simulink model "RFID"  (R2023a)
settings: Solver=VariableStepAuto  StartTime=0.0  StopTime=10.0  RelTol=1e-3
(part 1 of 2)
settings Model: Creator=SESA710169  LastModifiedBy=SESA710169

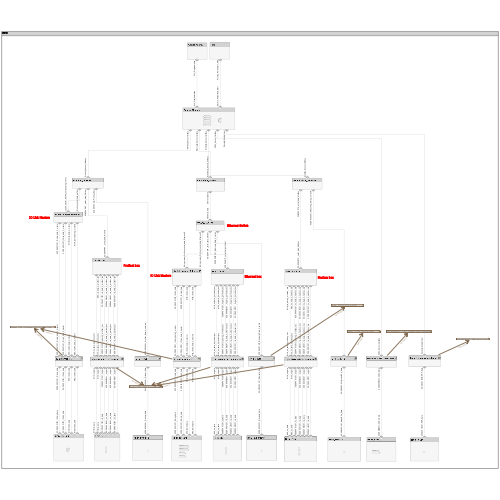
[thumbnail: Simulink's stored preview of the top-level diagram]
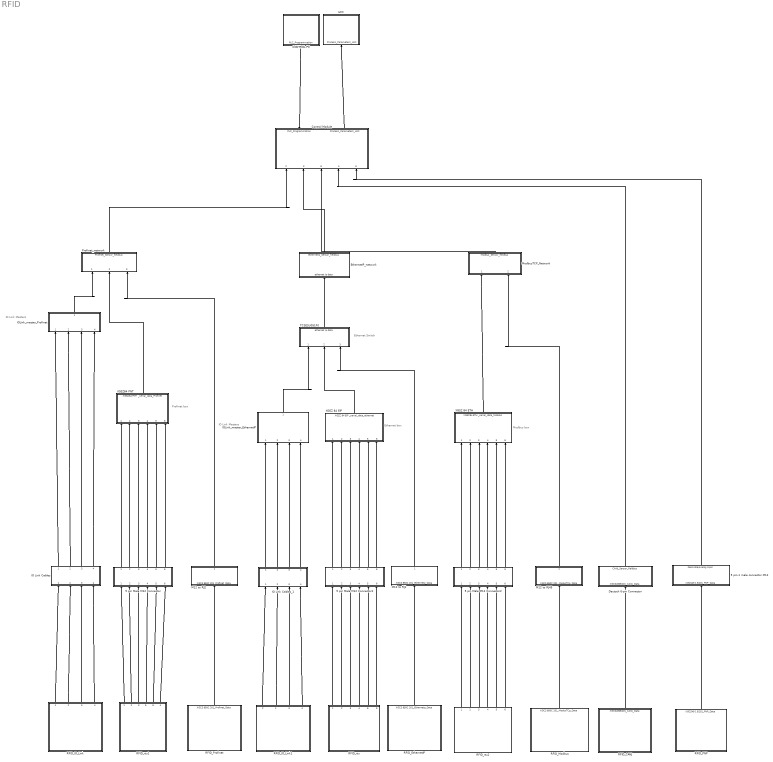
== system RFID ==
  note: IO Link Masters
  note: Modbus box
  note: Ethernet Switch
  note: Ethernet box
  note: IO Link Masters
  note: Profinet box
  5 pin Male M12 Connector : Subsystem
      settings: PortSchema="{\"entries\":[{\"content\":{\"headerSize\":26,\"margin\":15,\"minimumSpacing\":25,\"sides\":[{\"content\":{},\"type\":\"ConnectorPlacement.EquallySpacedRectSide\",\"uuid\":\"15872914-72ca-49c0-af57-e7ce3a34352d\"},{\"content\":{\"side\":\"RIGHT\"},\"type\":\"ConnectorPlacement.EquallySpacedRectSide\",\"uuid\":\"e1987595-5073-4cb0-bc3a-ce3e48eeeb38\"},{\"content\":{\"connectorIds\":[\"Out1\",\"Out2\",\"Out3\",\"Out4\",\"Out5\",\"Out6\"],\"side\":\"TOP\"},\"type\":\"ConnectorPlacement.EquallySpacedRectSide\",\"uuid\":\"34465e36-1a4b-47f4-80e2-40bdf2aa77c4\"},{\"content\":{\"connectorIds\":[\"In1\",\"In2\",\"In3\",\"In4\",\"In5\",\"In6\"],\"side\":\"BOTTOM\"},\"type\":\"ConnectorPlacement.EquallySpacedRectSide\",\"uuid\":\"7ee8196c-d26c-4fad-bba2-16755bce26d2\"}]},\"type\":\"ConnectorPlacement.EquallySpacedConnector\",\"uuid\":\"ac1f4730-dff7-48b7-9147-a46c79733028\"}],\"packageUris\":[\"http://schema.mathworks.com/mf0/Connector/R2020b\"],\"version\":\"1.0\"}"
  5 pin Male M12 Connector1 : Subsystem
      settings: PortSchema="{\"entries\":[{\"content\":{\"headerSize\":26,\"margin\":15,\"minimumSpacing\":25,\"sides\":[{\"content\":{},\"type\":\"ConnectorPlacement.EquallySpacedRectSide\",\"uuid\":\"15872914-72ca-49c0-af57-e7ce3a34352d\"},{\"content\":{\"side\":\"RIGHT\"},\"type\":\"ConnectorPlacement.EquallySpacedRectSide\",\"uuid\":\"e1987595-5073-4cb0-bc3a-ce3e48eeeb38\"},{\"content\":{\"connectorIds\":[\"Out1\",\"Out2\",\"Out3\",\"Out4\",\"Out5\",\"Out6\"],\"side\":\"TOP\"},\"type\":\"ConnectorPlacement.EquallySpacedRectSide\",\"uuid\":\"34465e36-1a4b-47f4-80e2-40bdf2aa77c4\"},{\"content\":{\"connectorIds\":[\"In1\",\"In2\",\"In3\",\"In4\",\"In5\",\"In6\"],\"side\":\"BOTTOM\"},\"type\":\"ConnectorPlacement.EquallySpacedRectSide\",\"uuid\":\"7ee8196c-d26c-4fad-bba2-16755bce26d2\"}]},\"type\":\"ConnectorPlacement.EquallySpacedConnector\",\"uuid\":\"ac1f4730-dff7-48b7-9147-a46c79733028\"}],\"packageUris\":[\"http://schema.mathworks.com/mf0/Connector/R2020b\"],\"version\":\"1.0\"}"
  5 pin Male M12 Connector2 : Subsystem
      settings: PortSchema="{\"entries\":[{\"content\":{\"headerSize\":26,\"margin\":15,\"minimumSpacing\":25,\"sides\":[{\"content\":{},\"type\":\"ConnectorPlacement.EquallySpacedRectSide\",\"uuid\":\"15872914-72ca-49c0-af57-e7ce3a34352d\"},{\"content\":{\"side\":\"RIGHT\"},\"type\":\"ConnectorPlacement.EquallySpacedRectSide\",\"uuid\":\"e1987595-5073-4cb0-bc3a-ce3e48eeeb38\"},{\"content\":{\"connectorIds\":[\"Out1\",\"Out2\",\"Out3\",\"Out4\",\"Out5\",\"Out6\"],\"side\":\"TOP\"},\"type\":\"ConnectorPlacement.EquallySpacedRectSide\",\"uuid\":\"34465e36-1a4b-47f4-80e2-40bdf2aa77c4\"},{\"content\":{\"connectorIds\":[\"In1\",\"In2\",\"In3\",\"In4\",\"In5\",\"In6\"],\"side\":\"BOTTOM\"},\"type\":\"ConnectorPlacement.EquallySpacedRectSide\",\"uuid\":\"7ee8196c-d26c-4fad-bba2-16755bce26d2\"}]},\"type\":\"ConnectorPlacement.EquallySpacedConnector\",\"uuid\":\"ac1f4730-dff7-48b7-9147-a46c79733028\"}],\"packageUris\":[\"http://schema.mathworks.com/mf0/Connector/R2020b\"],\"version\":\"1.0\"}"
  5 pin-1 male connector M12 : Subsystem
      settings: PortSchema="{\"entries\":[{\"content\":{\"headerSize\":26,\"margin\":15,\"minimumSpacing\":25,\"sides\":[{\"content\":{},\"type\":\"ConnectorPlacement.EquallySpacedRectSide\",\"uuid\":\"fd0e21b1-4690-476b-bc14-5c8fc71147f2\"},{\"content\":{\"side\":\"RIGHT\"},\"type\":\"ConnectorPlacement.EquallySpacedRectSide\",\"uuid\":\"81f5b1ef-d6a4-481c-8562-3dd4bbf12531\"},{\"content\":{\"connectorIds\":[\"Out1\"],\"side\":\"TOP\"},\"type\":\"ConnectorPlacement.EquallySpacedRectSide\",\"uuid\":\"ad97ad28-8845-419a-93af-6ade5c0bdfbe\"},{\"content\":{\"connectorIds\":[\"In1\"],\"side\":\"BOTTOM\"},\"type\":\"ConnectorPlacement.EquallySpacedRectSide\",\"uuid\":\"20c3ec93-f654-4080-81db-cffef7cb2cf6\"}]},\"type\":\"ConnectorPlacement.EquallySpacedConnector\",\"uuid\":\"3726fd7c-4b1c-4d15-a99a-e883e4d72662\"}],\"packageUris\":[\"http://schema.mathworks.com/mf0/Connector/R2020b\"],\"version\":\"1.0\"}"
  CONTROL PC : Subsystem
      settings: PortSchema="{\"entries\":[{\"content\":{\"headerSize\":26,\"margin\":15,\"minimumSpacing\":25,\"sides\":[{\"content\":{},\"type\":\"ConnectorPlacement.EquallySpacedRectSide\",\"uuid\":\"ff8f3bf2-d6f6-4ecc-9677-a0e5f5ade440\"},{\"content\":{\"side\":\"RIGHT\"},\"type\":\"ConnectorPlacement.EquallySpacedRectSide\",\"uuid\":\"fe155757-f3d5-40d8-a583-dbbc24843437\"},{\"content\":{\"side\":\"TOP\"},\"type\":\"ConnectorPlacement.EquallySpacedRectSide\",\"uuid\":\"51bc4fd0-0675-45de-93bd-0dc8d94c5489\"},{\"content\":{\"connectorIds\":[\"Out1\"],\"side\":\"BOTTOM\"},\"type\":\"ConnectorPlacement.EquallySpacedRectSide\",\"uuid\":\"d1c979f7-175f-4276-8069-5d6ac2f759ac\"}]},\"type\":\"ConnectorPlacement.EquallySpacedConnector\",\"uuid\":\"7eb8fdf8-dbe2-49f3-b9bd-384f85dcc997\"}],\"packageUris\":[\"http://schema.mathworks.com/mf0/Connector/R2020b\"],\"version\":\"1.0\"}"
  Control Module : Subsystem
      settings: PortSchema="{\"entries\":[{\"content\":{\"headerSize\":26,\"margin\":15,\"minimumSpacing\":25,\"sides\":[{\"content\":{},\"type\":\"ConnectorPlacement.EquallySpacedRectSide\",\"uuid\":\"1d52692e-0f44-4113-9236-a25bdb619ad6\"},{\"content\":{\"side\":\"RIGHT\"},\"type\":\"ConnectorPlacement.EquallySpacedRectSide\",\"uuid\":\"ebd7129d-6295-43a2-a8fa-ceade73e4712\"},{\"content\":{\"connectorIds\":[\"In1\",\"Out1\"],\"side\":\"TOP\"},\"type\":\"ConnectorPlacement.EquallySpacedRectSide\",\"uuid\":\"449c4e30-53b6-483f-ab84-235a0572996a\"},{\"content\":{\"connectorIds\":[\"In2\",\"In3\",\"In6\",\"In4\",\"In5\"],\"side\":\"BOTTOM\"},\"type\":\"ConnectorPlacement.EquallySpacedRectSide\",\"uuid\":\"9ddc23bf-eea9-4734-a916-f94a55c11bfe\"}]},\"type\":\"ConnectorPlacement.EquallySpacedConnector\",\"uuid\":\"d9df497a-181c-43b5-b6eb-3f69da1cdffc\"}],\"packageUris\":[\"http://schema.mathworks.com/mf0/Connector/R2020b\"],\"version\":\"1.0\"}"
  Deutsch 6-pin Connector : Subsystem
      settings: PortSchema="{\"entries\":[{\"content\":{\"headerSize\":26,\"margin\":15,\"minimumSpacing\":25,\"sides\":[{\"content\":{},\"type\":\"ConnectorPlacement.EquallySpacedRectSide\",\"uuid\":\"fd0e21b1-4690-476b-bc14-5c8fc71147f2\"},{\"content\":{\"side\":\"RIGHT\"},\"type\":\"ConnectorPlacement.EquallySpacedRectSide\",\"uuid\":\"81f5b1ef-d6a4-481c-8562-3dd4bbf12531\"},{\"content\":{\"connectorIds\":[\"Out1\"],\"side\":\"TOP\"},\"type\":\"ConnectorPlacement.EquallySpacedRectSide\",\"uuid\":\"ad97ad28-8845-419a-93af-6ade5c0bdfbe\"},{\"content\":{\"connectorIds\":[\"In1\"],\"side\":\"BOTTOM\"},\"type\":\"ConnectorPlacement.EquallySpacedRectSide\",\"uuid\":\"6cb1918c-498c-482e-975f-fc177a7f5f38\"}]},\"type\":\"ConnectorPlacement.EquallySpacedConnector\",\"uuid\":\"3726fd7c-4b1c-4d15-a99a-e883e4d72662\"}],\"packageUris\":[\"http://schema.mathworks.com/mf0/Connector/R2020b\"],\"version\":\"1.0\"}"
  EthernetIP_network : Subsystem
      settings: PortSchema="{\"entries\":[{\"content\":{\"headerSize\":26,\"margin\":15,\"minimumSpacing\":25,\"sides\":[{\"content\":{},\"type\":\"ConnectorPlacement.EquallySpacedRectSide\",\"uuid\":\"ff8f3bf2-d6f6-4ecc-9677-a0e5f5ade440\"},{\"content\":{\"side\":\"RIGHT\"},\"type\":\"ConnectorPlacement.EquallySpacedRectSide\",\"uuid\":\"fe155757-f3d5-40d8-a583-dbbc24843437\"},{\"content\":{\"connectorIds\":[\"Out1\"],\"side\":\"TOP\"},\"type\":\"ConnectorPlacement.EquallySpacedRectSide\",\"uuid\":\"51bc4fd0-0675-45de-93bd-0dc8d94c5489\"},{\"content\":{\"connectorIds\":[\"In1\"],\"side\":\"BOTTOM\"},\"type\":\"ConnectorPlacement.EquallySpacedRectSide\",\"uuid\":\"a6a48096-45e8-4078-827c-8af3dc9f1ee5\"}]},\"type\":\"ConnectorPlacement.EquallySpacedConnector\",\"uuid\":\"7eb8fdf8-dbe2-49f3-b9bd-384f85dcc997\"}],\"packageUris\":[\"http://schema.mathworks.com/mf0/Connector/R2020b\"],\"version\":\"1.0\"}"
  HMI : Subsystem
      settings: PortSchema="{\"entries\":[{\"content\":{\"headerSize\":26,\"margin\":15,\"minimumSpacing\":25,\"sides\":[{\"content\":{},\"type\":\"ConnectorPlacement.EquallySpacedRectSide\",\"uuid\":\"ff8f3bf2-d6f6-4ecc-9677-a0e5f5ade440\"},{\"content\":{\"side\":\"RIGHT\"},\"type\":\"ConnectorPlacement.EquallySpacedRectSide\",\"uuid\":\"fe155757-f3d5-40d8-a583-dbbc24843437\"},{\"content\":{\"side\":\"TOP\"},\"type\":\"ConnectorPlacement.EquallySpacedRectSide\",\"uuid\":\"51bc4fd0-0675-45de-93bd-0dc8d94c5489\"},{\"content\":{\"connectorIds\":[\"In1\"],\"side\":\"BOTTOM\"},\"type\":\"ConnectorPlacement.EquallySpacedRectSide\",\"uuid\":\"52c645db-393c-4514-a828-b3b130807567\"}]},\"type\":\"ConnectorPlacement.EquallySpacedConnector\",\"uuid\":\"7eb8fdf8-dbe2-49f3-b9bd-384f85dcc997\"}],\"packageUris\":[\"http://schema.mathworks.com/mf0/Connector/R2020b\"],\"version\":\"1.0\"}"
  IO Link Cables : Subsystem
      settings: PortSchema="{\"entries\":[{\"content\":{\"headerSize\":26,\"margin\":15,\"minimumSpacing\":25,\"sides\":[{\"content\":{},\"type\":\"ConnectorPlacement.EquallySpacedRectSide\",\"uuid\":\"114e0369-1e7a-4a46-bf9a-9a919302ecfe\"},{\"content\":{\"side\":\"RIGHT\"},\"type\":\"ConnectorPlacement.EquallySpacedRectSide\",\"uuid\":\"b401c2e5-2b5e-49de-abeb-2a7da0ded51e\"},{\"content\":{\"connectorIds\":[\"Out1\",\"Out2\",\"Out3\",\"Out4\"],\"side\":\"TOP\"},\"type\":\"ConnectorPlacement.EquallySpacedRectSide\",\"uuid\":\"300c240b-1dd5-4827-92ce-421815ba1fec\"},{\"content\":{\"connectorIds\":[\"In1\",\"In2\",\"In3\",\"In4\"],\"side\":\"BOTTOM\"},\"type\":\"ConnectorPlacement.EquallySpacedRectSide\",\"uuid\":\"4925845a-f056-46c0-9ec5-2efc31482337\"}]},\"type\":\"ConnectorPlacement.EquallySpacedConnector\",\"uuid\":\"3ba3c251-a23f-40e6-ae10-3e1f576377ed\"}],\"packageUris\":[\"http://schema.mathworks.com/mf0/Connector/R2020b\"],\"version\":\"1.0\"}"
  IO Link Cables_1 : Subsystem
      settings: PortSchema="{\"entries\":[{\"content\":{\"headerSize\":26,\"margin\":15,\"minimumSpacing\":25,\"sides\":[{\"content\":{},\"type\":\"ConnectorPlacement.EquallySpacedRectSide\",\"uuid\":\"114e0369-1e7a-4a46-bf9a-9a919302ecfe\"},{\"content\":{\"side\":\"RIGHT\"},\"type\":\"ConnectorPlacement.EquallySpacedRectSide\",\"uuid\":\"b401c2e5-2b5e-49de-abeb-2a7da0ded51e\"},{\"content\":{\"connectorIds\":[\"Out1\",\"Out2\",\"Out3\",\"Out4\"],\"side\":\"TOP\"},\"type\":\"ConnectorPlacement.EquallySpacedRectSide\",\"uuid\":\"300c240b-1dd5-4827-92ce-421815ba1fec\"},{\"content\":{\"connectorIds\":[\"In1\",\"In2\",\"In3\",\"In4\"],\"side\":\"BOTTOM\"},\"type\":\"ConnectorPlacement.EquallySpacedRectSide\",\"uuid\":\"4925845a-f056-46c0-9ec5-2efc31482337\"}]},\"type\":\"ConnectorPlacement.EquallySpacedConnector\",\"uuid\":\"3ba3c251-a23f-40e6-ae10-3e1f576377ed\"}],\"packageUris\":[\"http://schema.mathworks.com/mf0/Connector/R2020b\"],\"version\":\"1.0\"}"
  IOLink_master_EthernetIP : Subsystem
      settings: PortSchema="{\"entries\":[{\"content\":{\"headerSize\":26,\"margin\":15,\"minimumSpacing\":25,\"sides\":[{\"content\":{},\"type\":\"ConnectorPlacement.EquallySpacedRectSide\",\"uuid\":\"ff8f3bf2-d6f6-4ecc-9677-a0e5f5ade440\"},{\"content\":{\"side\":\"RIGHT\"},\"type\":\"ConnectorPlacement.EquallySpacedRectSide\",\"uuid\":\"fe155757-f3d5-40d8-a583-dbbc24843437\"},{\"content\":{\"connectorIds\":[\"Out1\"],\"side\":\"TOP\"},\"type\":\"ConnectorPlacement.EquallySpacedRectSide\",\"uuid\":\"51bc4fd0-0675-45de-93bd-0dc8d94c5489\"},{\"content\":{\"connectorIds\":[\"In1\",\"In2\",\"In3\",\"In4\"],\"side\":\"BOTTOM\"},\"type\":\"ConnectorPlacement.EquallySpacedRectSide\",\"uuid\":\"96d1ea42-fb86-44af-b869-0fda48dfe9a2\"}]},\"type\":\"ConnectorPlacement.EquallySpacedConnector\",\"uuid\":\"7eb8fdf8-dbe2-49f3-b9bd-384f85dcc997\"}],\"packageUris\":[\"http://schema.mathworks.com/mf0/Connector/R2020b\"],\"version\":\"1.0\"}"
  IOLink_master_Profinet : Subsystem
      settings: PortSchema="{\"entries\":[{\"content\":{\"headerSize\":26,\"margin\":15,\"minimumSpacing\":25,\"sides\":[{\"content\":{},\"type\":\"ConnectorPlacement.EquallySpacedRectSide\",\"uuid\":\"ff8f3bf2-d6f6-4ecc-9677-a0e5f5ade440\"},{\"content\":{\"side\":\"RIGHT\"},\"type\":\"ConnectorPlacement.EquallySpacedRectSide\",\"uuid\":\"fe155757-f3d5-40d8-a583-dbbc24843437\"},{\"content\":{\"connectorIds\":[\"Out1\"],\"side\":\"TOP\"},\"type\":\"ConnectorPlacement.EquallySpacedRectSide\",\"uuid\":\"51bc4fd0-0675-45de-93bd-0dc8d94c5489\"},{\"content\":{\"connectorIds\":[\"In1\",\"In2\",\"In3\",\"In4\"],\"side\":\"BOTTOM\"},\"type\":\"ConnectorPlacement.EquallySpacedRectSide\",\"uuid\":\"96d1ea42-fb86-44af-b869-0fda48dfe9a2\"}]},\"type\":\"ConnectorPlacement.EquallySpacedConnector\",\"uuid\":\"7eb8fdf8-dbe2-49f3-b9bd-384f85dcc997\"}],\"packageUris\":[\"http://schema.mathworks.com/mf0/Connector/R2020b\"],\"version\":\"1.0\"}"
  M12 to RJ1 : Subsystem
      settings: PortSchema="{\"entries\":[{\"content\":{\"headerSize\":26,\"margin\":15,\"minimumSpacing\":25,\"sides\":[{\"content\":{},\"type\":\"ConnectorPlacement.EquallySpacedRectSide\",\"uuid\":\"15872914-72ca-49c0-af57-e7ce3a34352d\"},{\"content\":{\"side\":\"RIGHT\"},\"type\":\"ConnectorPlacement.EquallySpacedRectSide\",\"uuid\":\"e1987595-5073-4cb0-bc3a-ce3e48eeeb38\"},{\"content\":{\"connectorIds\":[\"Out1\"],\"side\":\"TOP\"},\"type\":\"ConnectorPlacement.EquallySpacedRectSide\",\"uuid\":\"34465e36-1a4b-47f4-80e2-40bdf2aa77c4\"},{\"content\":{\"connectorIds\":[\"In1\"],\"side\":\"BOTTOM\"},\"type\":\"ConnectorPlacement.EquallySpacedRectSide\",\"uuid\":\"232f6760-6a21-49f2-ae01-222b23a991b9\"}]},\"type\":\"ConnectorPlacement.EquallySpacedConnector\",\"uuid\":\"ac1f4730-dff7-48b7-9147-a46c79733028\"}],\"packageUris\":[\"http://schema.mathworks.com/mf0/Connector/R2020b\"],\"version\":\"1.0\"}"
  M12 to RJ2 : Subsystem
      settings: PortSchema="{\"entries\":[{\"content\":{\"headerSize\":26,\"margin\":15,\"minimumSpacing\":25,\"sides\":[{\"content\":{},\"type\":\"ConnectorPlacement.EquallySpacedRectSide\",\"uuid\":\"15872914-72ca-49c0-af57-e7ce3a34352d\"},{\"content\":{\"side\":\"RIGHT\"},\"type\":\"ConnectorPlacement.EquallySpacedRectSide\",\"uuid\":\"e1987595-5073-4cb0-bc3a-ce3e48eeeb38\"},{\"content\":{\"connectorIds\":[\"Out1\"],\"side\":\"TOP\"},\"type\":\"ConnectorPlacement.EquallySpacedRectSide\",\"uuid\":\"34465e36-1a4b-47f4-80e2-40bdf2aa77c4\"},{\"content\":{\"connectorIds\":[\"In1\"],\"side\":\"BOTTOM\"},\"type\":\"ConnectorPlacement.EquallySpacedRectSide\",\"uuid\":\"232f6760-6a21-49f2-ae01-222b23a991b9\"}]},\"type\":\"ConnectorPlacement.EquallySpacedConnector\",\"uuid\":\"ac1f4730-dff7-48b7-9147-a46c79733028\"}],\"packageUris\":[\"http://schema.mathworks.com/mf0/Connector/R2020b\"],\"version\":\"1.0\"}"
  M12 to RJ45 : Subsystem
      settings: PortSchema="{\"entries\":[{\"content\":{\"headerSize\":26,\"margin\":15,\"minimumSpacing\":25,\"sides\":[{\"content\":{},\"type\":\"ConnectorPlacement.EquallySpacedRectSide\",\"uuid\":\"15872914-72ca-49c0-af57-e7ce3a34352d\"},{\"content\":{\"side\":\"RIGHT\"},\"type\":\"ConnectorPlacement.EquallySpacedRectSide\",\"uuid\":\"e1987595-5073-4cb0-bc3a-ce3e48eeeb38\"},{\"content\":{\"connectorIds\":[\"Out1\"],\"side\":\"TOP\"},\"type\":\"ConnectorPlacement.EquallySpacedRectSide\",\"uuid\":\"34465e36-1a4b-47f4-80e2-40bdf2aa77c4\"},{\"content\":{\"connectorIds\":[\"In1\"],\"side\":\"BOTTOM\"},\"type\":\"ConnectorPlacement.EquallySpacedRectSide\",\"uuid\":\"232f6760-6a21-49f2-ae01-222b23a991b9\"}]},\"type\":\"ConnectorPlacement.EquallySpacedConnector\",\"uuid\":\"ac1f4730-dff7-48b7-9147-a46c79733028\"}],\"packageUris\":[\"http://schema.mathworks.com/mf0/Connector/R2020b\"],\"version\":\"1.0\"}"
  ModbusTCP_Network : Subsystem
      settings: PortSchema="{\"entries\":[{\"content\":{\"headerSize\":26,\"margin\":15,\"minimumSpacing\":25,\"sides\":[{\"content\":{},\"type\":\"ConnectorPlacement.EquallySpacedRectSide\",\"uuid\":\"ff8f3bf2-d6f6-4ecc-9677-a0e5f5ade440\"},{\"content\":{\"side\":\"RIGHT\"},\"type\":\"ConnectorPlacement.EquallySpacedRectSide\",\"uuid\":\"fe155757-f3d5-40d8-a583-dbbc24843437\"},{\"content\":{\"connectorIds\":[\"Out1\"],\"side\":\"TOP\"},\"type\":\"ConnectorPlacement.EquallySpacedRectSide\",\"uuid\":\"51bc4fd0-0675-45de-93bd-0dc8d94c5489\"},{\"content\":{\"connectorIds\":[\"In1\",\"In2\"],\"side\":\"BOTTOM\"},\"type\":\"ConnectorPlacement.EquallySpacedRectSide\",\"uuid\":\"a6a48096-45e8-4078-827c-8af3dc9f1ee5\"}]},\"type\":\"ConnectorPlacement.EquallySpacedConnector\",\"uuid\":\"7eb8fdf8-dbe2-49f3-b9bd-384f85dcc997\"}],\"packageUris\":[\"http://schema.mathworks.com/mf0/Connector/R2020b\"],\"version\":\"1.0\"}"
  Profinet_network : Subsystem
      settings: PortSchema="{\"entries\":[{\"content\":{\"headerSize\":26,\"margin\":15,\"minimumSpacing\":25,\"sides\":[{\"content\":{},\"type\":\"ConnectorPlacement.EquallySpacedRectSide\",\"uuid\":\"ff8f3bf2-d6f6-4ecc-9677-a0e5f5ade440\"},{\"content\":{\"side\":\"RIGHT\"},\"type\":\"ConnectorPlacement.EquallySpacedRectSide\",\"uuid\":\"fe155757-f3d5-40d8-a583-dbbc24843437\"},{\"content\":{\"connectorIds\":[\"Out1\"],\"side\":\"TOP\"},\"type\":\"ConnectorPlacement.EquallySpacedRectSide\",\"uuid\":\"51bc4fd0-0675-45de-93bd-0dc8d94c5489\"},{\"content\":{\"connectorIds\":[\"In1\",\"In2\",\"In3\"],\"side\":\"BOTTOM\"},\"type\":\"ConnectorPlacement.EquallySpacedRectSide\",\"uuid\":\"a6a48096-45e8-4078-827c-8af3dc9f1ee5\"}]},\"type\":\"ConnectorPlacement.EquallySpacedConnector\",\"uuid\":\"7eb8fdf8-dbe2-49f3-b9bd-384f85dcc997\"}],\"packageUris\":[\"http://schema.mathworks.com/mf0/Connector/R2020b\"],\"version\":\"1.0\"}"
  RFID_CANJ : Subsystem
      settings: PortSchema="{\"entries\":[{\"content\":{\"headerSize\":26,\"margin\":15,\"minimumSpacing\":25,\"sides\":[{\"content\":{},\"type\":\"ConnectorPlacement.EquallySpacedRectSide\",\"uuid\":\"e0eb1e50-4962-459a-8fec-1c017d32fce9\"},{\"content\":{\"side\":\"RIGHT\"},\"type\":\"ConnectorPlacement.EquallySpacedRectSide\",\"uuid\":\"13b866c0-40d0-4daf-b8cf-e6d1decf5d11\"},{\"content\":{\"connectorIds\":[\"Out1\"],\"side\":\"TOP\"},\"type\":\"ConnectorPlacement.EquallySpacedRectSide\",\"uuid\":\"2f503909-3154-427d-b557-3b7bc001611f\"}]},\"type\":\"ConnectorPlacement.EquallySpacedConnector\",\"uuid\":\"e4954000-e918-49fc-93eb-b443de9c48d9\"}],\"packageUris\":[\"http://schema.mathworks.com/mf0/Connector/R2020b\"],\"version\":\"1.0\"}"
  RFID_EthernetIP : Subsystem
      settings: PortSchema="{\"entries\":[{\"content\":{\"headerSize\":26,\"margin\":15,\"minimumSpacing\":25,\"sides\":[{\"content\":{},\"type\":\"ConnectorPlacement.EquallySpacedRectSide\",\"uuid\":\"e0eb1e50-4962-459a-8fec-1c017d32fce9\"},{\"content\":{\"side\":\"RIGHT\"},\"type\":\"ConnectorPlacement.EquallySpacedRectSide\",\"uuid\":\"13b866c0-40d0-4daf-b8cf-e6d1decf5d11\"},{\"content\":{\"connectorIds\":[\"Out1\"],\"side\":\"TOP\"},\"type\":\"ConnectorPlacement.EquallySpacedRectSide\",\"uuid\":\"2f503909-3154-427d-b557-3b7bc001611f\"}]},\"type\":\"ConnectorPlacement.EquallySpacedConnector\",\"uuid\":\"e4954000-e918-49fc-93eb-b443de9c48d9\"}],\"packageUris\":[\"http://schema.mathworks.com/mf0/Connector/R2020b\"],\"version\":\"1.0\"}"
  RFID_IO_Link : Subsystem
      settings: PortSchema="{\"entries\":[{\"content\":{\"headerSize\":26,\"margin\":15,\"minimumSpacing\":25,\"sides\":[{\"content\":{},\"type\":\"ConnectorPlacement.EquallySpacedRectSide\",\"uuid\":\"ff8f3bf2-d6f6-4ecc-9677-a0e5f5ade440\"},{\"content\":{\"side\":\"RIGHT\"},\"type\":\"ConnectorPlacement.EquallySpacedRectSide\",\"uuid\":\"fe155757-f3d5-40d8-a583-dbbc24843437\"},{\"content\":{\"connectorIds\":[\"Out1\",\"Out2\",\"Out3\",\"Out4\"],\"side\":\"TOP\"},\"type\":\"ConnectorPlacement.EquallySpacedRectSide\",\"uuid\":\"51bc4fd0-0675-45de-93bd-0dc8d94c5489\"}]},\"type\":\"ConnectorPlacement.EquallySpacedConnector\",\"uuid\":\"7eb8fdf8-dbe2-49f3-b9bd-384f85dcc997\"}],\"packageUris\":[\"http://schema.mathworks.com/mf0/Connector/R2020b\"],\"version\":\"1.0\"}"
  RFID_IO_Link1 : Subsystem
      settings: PortSchema="{\"entries\":[{\"content\":{\"headerSize\":26,\"margin\":15,\"minimumSpacing\":25,\"sides\":[{\"content\":{},\"type\":\"ConnectorPlacement.EquallySpacedRectSide\",\"uuid\":\"ff8f3bf2-d6f6-4ecc-9677-a0e5f5ade440\"},{\"content\":{\"side\":\"RIGHT\"},\"type\":\"ConnectorPlacement.EquallySpacedRectSide\",\"uuid\":\"fe155757-f3d5-40d8-a583-dbbc24843437\"},{\"content\":{\"connectorIds\":[\"Out2\",\"Out1\",\"Out3\",\"Out4\"],\"side\":\"TOP\"},\"type\":\"ConnectorPlacement.EquallySpacedRectSide\",\"uuid\":\"51bc4fd0-0675-45de-93bd-0dc8d94c5489\"}]},\"type\":\"ConnectorPlacement.EquallySpacedConnector\",\"uuid\":\"7eb8fdf8-dbe2-49f3-b9bd-384f85dcc997\"}],\"packageUris\":[\"http://schema.mathworks.com/mf0/Connector/R2020b\"],\"version\":\"1.0\"}"
  RFID_Modbus : Subsystem
      settings: PortSchema="{\"entries\":[{\"content\":{\"headerSize\":26,\"margin\":15,\"minimumSpacing\":25,\"sides\":[{\"content\":{},\"type\":\"ConnectorPlacement.EquallySpacedRectSide\",\"uuid\":\"e0eb1e50-4962-459a-8fec-1c017d32fce9\"},{\"content\":{\"side\":\"RIGHT\"},\"type\":\"ConnectorPlacement.EquallySpacedRectSide\",\"uuid\":\"13b866c0-40d0-4daf-b8cf-e6d1decf5d11\"},{\"content\":{\"connectorIds\":[\"Out1\"],\"side\":\"TOP\"},\"type\":\"ConnectorPlacement.EquallySpacedRectSide\",\"uuid\":\"2f503909-3154-427d-b557-3b7bc001611f\"}]},\"type\":\"ConnectorPlacement.EquallySpacedConnector\",\"uuid\":\"e4954000-e918-49fc-93eb-b443de9c48d9\"}],\"packageUris\":[\"http://schema.mathworks.com/mf0/Connector/R2020b\"],\"version\":\"1.0\"}"
  RFID_PNP : Subsystem
      settings: PortSchema="{\"entries\":[{\"content\":{\"headerSize\":26,\"margin\":15,\"minimumSpacing\":25,\"sides\":[{\"content\":{},\"type\":\"ConnectorPlacement.EquallySpacedRectSide\",\"uuid\":\"e0eb1e50-4962-459a-8fec-1c017d32fce9\"},{\"content\":{\"side\":\"RIGHT\"},\"type\":\"ConnectorPlacement.EquallySpacedRectSide\",\"uuid\":\"13b866c0-40d0-4daf-b8cf-e6d1decf5d11\"},{\"content\":{\"connectorIds\":[\"Out1\"],\"side\":\"TOP\"},\"type\":\"ConnectorPlacement.EquallySpacedRectSide\",\"uuid\":\"2f503909-3154-427d-b557-3b7bc001611f\"}]},\"type\":\"ConnectorPlacement.EquallySpacedConnector\",\"uuid\":\"e4954000-e918-49fc-93eb-b443de9c48d9\"}],\"packageUris\":[\"http://schema.mathworks.com/mf0/Connector/R2020b\"],\"version\":\"1.0\"}"
  RFID_Profinet : Subsystem
      settings: PortSchema="{\"entries\":[{\"content\":{\"headerSize\":26,\"margin\":15,\"minimumSpacing\":25,\"sides\":[{\"content\":{},\"type\":\"ConnectorPlacement.EquallySpacedRectSide\",\"uuid\":\"e0eb1e50-4962-459a-8fec-1c017d32fce9\"},{\"content\":{\"side\":\"RIGHT\"},\"type\":\"ConnectorPlacement.EquallySpacedRectSide\",\"uuid\":\"13b866c0-40d0-4daf-b8cf-e6d1decf5d11\"},{\"content\":{\"connectorIds\":[\"Out1\"],\"side\":\"TOP\"},\"type\":\"ConnectorPlacement.EquallySpacedRectSide\",\"uuid\":\"2f503909-3154-427d-b557-3b7bc001611f\"}]},\"type\":\"ConnectorPlacement.EquallySpacedConnector\",\"uuid\":\"e4954000-e918-49fc-93eb-b443de9c48d9\"}],\"packageUris\":[\"http://schema.mathworks.com/mf0/Connector/R2020b\"],\"version\":\"1.0\"}"
  RFID_rtu : Subsystem
      settings: PortSchema="{\"entries\":[{\"content\":{\"headerSize\":26,\"margin\":15,\"minimumSpacing\":25,\"sides\":[{\"content\":{},\"type\":\"ConnectorPlacement.EquallySpacedRectSide\",\"uuid\":\"e0eb1e50-4962-459a-8fec-1c017d32fce9\"},{\"content\":{\"side\":\"RIGHT\"},\"type\":\"ConnectorPlacement.EquallySpacedRectSide\",\"uuid\":\"13b866c0-40d0-4daf-b8cf-e6d1decf5d11\"},{\"content\":{\"connectorIds\":[\"Out1\",\"Out2\",\"Out3\",\"Out4\",\"Out6\",\"Out5\"],\"side\":\"TOP\"},\"type\":\"ConnectorPlacement.EquallySpacedRectSide\",\"uuid\":\"2f503909-3154-427d-b557-3b7bc001611f\"}]},\"type\":\"ConnectorPlacement.EquallySpacedConnector\",\"uuid\":\"e4954000-e918-49fc-93eb-b443de9c48d9\"}],\"packageUris\":[\"http://schema.mathworks.com/mf0/Connector/R2020b\"],\"version\":\"1.0\"}"
  RFID_rtu1 : Subsystem
      settings: PortSchema="{\"entries\":[{\"content\":{\"headerSize\":26,\"margin\":15,\"minimumSpacing\":25,\"sides\":[{\"content\":{},\"type\":\"ConnectorPlacement.EquallySpacedRectSide\",\"uuid\":\"e0eb1e50-4962-459a-8fec-1c017d32fce9\"},{\"content\":{\"side\":\"RIGHT\"},\"type\":\"ConnectorPlacement.EquallySpacedRectSide\",\"uuid\":\"13b866c0-40d0-4daf-b8cf-e6d1decf5d11\"},{\"content\":{\"connectorIds\":[\"Out1\",\"Out2\",\"Out3\",\"Out5\",\"Out6\",\"Out4\"],\"side\":\"TOP\"},\"type\":\"ConnectorPlacement.EquallySpacedRectSide\",\"uuid\":\"2f503909-3154-427d-b557-3b7bc001611f\"}]},\"type\":\"ConnectorPlacement.EquallySpacedConnector\",\"uuid\":\"e4954000-e918-49fc-93eb-b443de9c48d9\"}],\"packageUris\":[\"http://schema.mathworks.com/mf0/Connector/R2020b\"],\"version\":\"1.0\"}"
  RFID_rtu2 : Subsystem
      settings: PortSchema="{\"entries\":[{\"content\":{\"headerSize\":26,\"margin\":15,\"minimumSpacing\":25,\"sides\":[{\"content\":{},\"type\":\"ConnectorPlacement.EquallySpacedRectSide\",\"uuid\":\"e0eb1e50-4962-459a-8fec-1c017d32fce9\"},{\"content\":{\"side\":\"RIGHT\"},\"type\":\"ConnectorPlacement.EquallySpacedRectSide\",\"uuid\":\"13b866c0-40d0-4daf-b8cf-e6d1decf5d11\"},{\"content\":{\"connectorIds\":[\"Out1\",\"Out2\",\"Out3\",\"Out4\",\"Out5\",\"Out6\"],\"side\":\"TOP\"},\"type\":\"ConnectorPlacement.EquallySpacedRectSide\",\"uuid\":\"2f503909-3154-427d-b557-3b7bc001611f\"}]},\"type\":\"ConnectorPlacement.EquallySpacedConnector\",\"uuid\":\"e4954000-e918-49fc-93eb-b443de9c48d9\"}],\"packageUris\":[\"http://schema.mathworks.com/mf0/Connector/R2020b\"],\"version\":\"1.0\"}"
  TCSESU051F0 : Subsystem  Description=|
      | unmanaged Ethernet switch - 5 M12 copper ports - IP67
      | https://www.se.com/fr/fr/product/TCSESU051F0/switch-ethernet-non-manag%C3%A9-5-ports-cuivre-m12-ip67/
      settings: PortSchema="{\"entries\":[{\"content\":{\"headerSize\":26,\"margin\":15,\"minimumSpacing\":25,\"sides\":[{\"content\":{},\"type\":\"ConnectorPlacement.EquallySpacedRectSide\",\"uuid\":\"ff8f3bf2-d6f6-4ecc-9677-a0e5f5ade440\"},{\"content\":{\"side\":\"RIGHT\"},\"type\":\"ConnectorPlacement.EquallySpacedRectSide\",\"uuid\":\"fe155757-f3d5-40d8-a583-dbbc24843437\"},{\"content\":{\"connectorIds\":[\"Out1\"],\"side\":\"TOP\"},\"type\":\"ConnectorPlacement.EquallySpacedRectSide\",\"uuid\":\"51bc4fd0-0675-45de-93bd-0dc8d94c5489\"},{\"content\":{\"connectorIds\":[\"In1\",\"In2\",\"In3\"],\"side\":\"BOTTOM\"},\"type\":\"ConnectorPlacement.EquallySpacedRectSide\",\"uuid\":\"b60d271e-a2b5-4b89-880e-0cab92ae5cf5\"}]},\"type\":\"ConnectorPlacement.EquallySpacedConnector\",\"uuid\":\"7eb8fdf8-dbe2-49f3-b9bd-384f85dcc997\"}],\"packageUris\":[\"http://schema.mathworks.com/mf0/Connector/R2020b\"],\"version\":\"1.0\"}"
  "XGSZ 84 EIP " : Subsystem
      settings: PortSchema="{\"entries\":[{\"content\":{\"headerSize\":26,\"margin\":15,\"minimumSpacing\":25,\"sides\":[{\"content\":{},\"type\":\"ConnectorPlacement.EquallySpacedRectSide\",\"uuid\":\"ff8f3bf2-d6f6-4ecc-9677-a0e5f5ade440\"},{\"content\":{\"side\":\"RIGHT\"},\"type\":\"ConnectorPlacement.EquallySpacedRectSide\",\"uuid\":\"fe155757-f3d5-40d8-a583-dbbc24843437\"},{\"content\":{\"connectorIds\":[\"Out1\"],\"side\":\"TOP\"},\"type\":\"ConnectorPlacement.EquallySpacedRectSide\",\"uuid\":\"51bc4fd0-0675-45de-93bd-0dc8d94c5489\"},{\"content\":{\"connectorIds\":[\"In1\",\"In2\",\"In3\",\"In4\",\"In5\",\"In6\"],\"side\":\"BOTTOM\"},\"type\":\"ConnectorPlacement.EquallySpacedRectSide\",\"uuid\":\"6d197186-f4d0-493a-8e40-71ff05ce5da3\"}]},\"type\":\"ConnectorPlacement.EquallySpacedConnector\",\"uuid\":\"7eb8fdf8-dbe2-49f3-b9bd-384f85dcc997\"}],\"packageUris\":[\"http://schema.mathworks.com/mf0/Connector/R2020b\"],\"version\":\"1.0\"}"
  "XGSZ 84 ETH " : Subsystem
      settings: PortSchema="{\"entries\":[{\"content\":{\"headerSize\":26,\"margin\":15,\"minimumSpacing\":25,\"sides\":[{\"content\":{},\"type\":\"ConnectorPlacement.EquallySpacedRectSide\",\"uuid\":\"ff8f3bf2-d6f6-4ecc-9677-a0e5f5ade440\"},{\"content\":{\"side\":\"RIGHT\"},\"type\":\"ConnectorPlacement.EquallySpacedRectSide\",\"uuid\":\"fe155757-f3d5-40d8-a583-dbbc24843437\"},{\"content\":{\"connectorIds\":[\"Out1\"],\"side\":\"TOP\"},\"type\":\"ConnectorPlacement.EquallySpacedRectSide\",\"uuid\":\"51bc4fd0-0675-45de-93bd-0dc8d94c5489\"},{\"content\":{\"connectorIds\":[\"In1\",\"In2\",\"In3\",\"In4\",\"In5\",\"In6\"],\"side\":\"BOTTOM\"},\"type\":\"ConnectorPlacement.EquallySpacedRectSide\",\"uuid\":\"49ad1726-0f8f-4ceb-a395-70032c197de9\"}]},\"type\":\"ConnectorPlacement.EquallySpacedConnector\",\"uuid\":\"7eb8fdf8-dbe2-49f3-b9bd-384f85dcc997\"}],\"packageUris\":[\"http://schema.mathworks.com/mf0/Connector/R2020b\"],\"version\":\"1.0\"}"
  "XGSZ84 PNT " : Subsystem
      settings: PortSchema="{\"entries\":[{\"content\":{\"headerSize\":26,\"margin\":15,\"minimumSpacing\":25,\"sides\":[{\"content\":{},\"type\":\"ConnectorPlacement.EquallySpacedRectSide\",\"uuid\":\"ff8f3bf2-d6f6-4ecc-9677-a0e5f5ade440\"},{\"content\":{\"side\":\"RIGHT\"},\"type\":\"ConnectorPlacement.EquallySpacedRectSide\",\"uuid\":\"fe155757-f3d5-40d8-a583-dbbc24843437\"},{\"content\":{\"connectorIds\":[\"Out1\"],\"side\":\"TOP\"},\"type\":\"ConnectorPlacement.EquallySpacedRectSide\",\"uuid\":\"51bc4fd0-0675-45de-93bd-0dc8d94c5489\"},{\"content\":{\"connectorIds\":[\"In1\",\"In2\",\"In3\",\"In4\",\"In5\",\"In6\"],\"side\":\"BOTTOM\"},\"type\":\"ConnectorPlacement.EquallySpacedRectSide\",\"uuid\":\"1adba72b-967b-42d2-a1a0-4bd6f0d21c60\"}]},\"type\":\"ConnectorPlacement.EquallySpacedConnector\",\"uuid\":\"7eb8fdf8-dbe2-49f3-b9bd-384f85dcc997\"}],\"packageUris\":[\"http://schema.mathworks.com/mf0/Connector/R2020b\"],\"version\":\"1.0\"}"
  wires:
  TCSESU051F0/1(ethernet ip data) -> EthernetIP_network/1(ethernet ip data)
  "XGSZ 84 ETH "/1(XGSZ84 ETH _serial_data_Mobdus) -> ModbusTCP_Network/1(XGSZ84 ETH _serial_data_Mobdus)
  "XGSZ84 PNT "/1(XGSZ84 PNT  _serial_data_Profinet) -> Profinet_network/2(XGSZ84 PNT  _serial_data_Profinet)
  IOLink_master_Profinet/1(IOLink_master_Profinet_serial_data_profinet) -> Profinet_network/1(IOLink_master_Profinet_serial_data_profinet)
  "XGSZ 84 EIP "/1(XGSZ 84 EIP _serial_data_ethernet) -> TCSESU051F0/2(XGSZ 84 EIP _serial_data_ethernet)
  IOLink_master_EthernetIP/1(IOLink_master_Profinet_serial_data_EthernetIP) -> TCSESU051F0/1(IOLink_master_Profinet_serial_data_EthernetIP)
  RFID_EthernetIP/1(XGCS 850C 201_Ethernetp_Data) -> M12 to RJ1/1(XGCS 850C 201_Ethernetp_Data)
  CONTROL PC/1(PLC_Programmation) -> Control Module/1(PLC_Programmation)
  Profinet_network/1(Profinet_Sensor_fieldbus) -> Control Module/2(Profinet_Sensor_fieldbus)
  EthernetIP_network/1(Ethernetip_Sensor_fieldbus) -> Control Module/3(Ethernetip_Sensor_fieldbus)
  ModbusTCP_Network/1(Modbus_Sensor_fieldbus) -> Control Module/6(Modbus_Sensor_fieldbus)
  Control Module/1(Process_Parameters_HMI) -> HMI/1(Process_Parameters_HMI)
  RFID_PNP/1(XGCS49 1 B201_PNP_Data) -> 5 pin-1 male connector M12/1(XGCS49 1 B201_PNP_Data)
  5 pin-1 male connector M12/1(Descrete/Analog Input) -> Control Module/5(Descrete/Analog Input)
  RFID_CANJ/1(XGCS460B201_CANJ_Data) -> Deutsch 6-pin Connector/1(XGCS460B201_CANJ_Data)
  Deutsch 6-pin Connector/1(CANJ_Sensor_fieldbus) -> Control Module/4(CANJ_Sensor_fieldbus)
  RFID_IO_Link/1(XGCS 89 01201_IOLimk_data) -> IO Link Cables/1(XGCS 89 01201_IOLimk_data)
  IO Link Cables/1(XGCS 89 01201_IOLimk_data_2_master) -> IOLink_master_Profinet/1(XGCS 89 01201_IOLimk_data_2_master)
  RFID_IO_Link/2(XGCS 49 01201_IOLink_data) -> IO Link Cables/2(XGCS 49 01201_IOLink_data)
  RFID_IO_Link/3(M18_IOLink_data) -> IO Link Cables/3(M18_IOLink_data)
  RFID_IO_Link/4(M30_IOLink_data) -> IO Link Cables/4(M30_IOLink_data)
  IO Link Cables/2(XGCS 49 01201_IOLink_data_2_master) -> IOLink_master_Profinet/2(XGCS 49 01201_IOLink_data_2_master)
  IO Link Cables/3(M18_IOLink_data_2_master) -> IOLink_master_Profinet/3(M18_IOLink_data_2_master)
  IO Link Cables/4(M30_IOLink_data_2_masters) -> IOLink_master_Profinet/4(M30_IOLink_data_2_masters)
  RFID_IO_Link1/2(XGCS 49 01201_IOLink_data) -> IO Link Cables_1/1(XGCS 89 01201_IOLimk_data)
  IO Link Cables_1/1(XGCS 89 01201_IOLimk_data_2_master) -> IOLink_master_EthernetIP/1(XGCS 49 01201_IOLink_data)
  IO Link Cables_1/2(XGCS 49 01201_IOLink_data_2_master) -> IOLink_master_EthernetIP/2(XGCS 89 01201_IOLimk_data)
  IO Link Cables_1/3(M18_IOLink_data_2_master) -> IOLink_master_EthernetIP/3(M18_IOLink_data)
  IO Link Cables_1/4(M30_IOLink_data_2_masters) -> IOLink_master_EthernetIP/4(M30_IOLink_data)
  RFID_IO_Link1/1(XGCS 89 01201_IOLimk_data) -> IO Link Cables_1/2(XGCS 49 01201_IOLink_data)
  RFID_IO_Link1/3(M18_IOLink_data) -> IO Link Cables_1/3(M18_IOLink_data)
  RFID_IO_Link1/4(M30_IOLink_data) -> IO Link Cables_1/4(M30_IOLink_data)
  RFID_rtu1/1(M18_rtu_data) -> 5 pin Male M12 Connector/1(M18_rtu_data)
  RFID_rtu1/2(M30_rtu_data) -> 5 pin Male M12 Connector/2(M30_rtu_data)
  RFID_rtu1/3(XGCS49 0 1201_rtu_data) -> 5 pin Male M12 Connector/3(XGCS49 0 1201_rtu_data)
  RFID_rtu1/5(XGCS49 0 B201 _rtu_data) -> 5 pin Male M12 Connector/4(XGCS49 0 B201 _rtu_data)
  RFID_rtu1/6(XGCS49 L B201 _rtu_data) -> 5 pin Male M12 Connector/5(XGCS49 L B201 _rtu_data)
  RFID_rtu1/4(XGCS 89 01201 _rtu_data) -> 5 pin Male M12 Connector/6(XGCS 89 01201 _rtu_data)
  5 pin Male M12 Connector/1(M18_rtu_data_2_profinet_box) -> "XGSZ84 PNT "/1(" ")
  5 pin Male M12 Connector/2(M30_rtu_data_2_profinet_box) -> "XGSZ84 PNT "/2(M30_rtu_data_2_profinet_box)
  5 pin Male M12 Connector/3(XGCS49 0 1201_rtu_data_2_profinet_box) -> "XGSZ84 PNT "/3(XGCS49 0 1201_rtu_data_2_profinet_box)
  5 pin Male M12 Connector/4(XGCS49 0 B201 _rtu_data_2_profinet_box) -> "XGSZ84 PNT "/4(XGCS49 0 B201 _rtu_data_2_profinet_box)
  5 pin Male M12 Connector/5(XGCS49 L B201 _rtu_data_2_profinet_box) -> "XGSZ84 PNT "/5(XGCS49 L B201 _rtu_data_2_profinet_box)
  5 pin Male M12 Connector/6(XGCS 89 01201 _rtu_data_2_profinet_box) -> "XGSZ84 PNT "/6(XGCS 89 01201 _rtu_data_2_profinet_box)
  RFID_rtu/1(M18_rtu_data) -> 5 pin Male M12 Connector1/1(M18_rtu_data)
  RFID_rtu/2(M30_rtu_data) -> 5 pin Male M12 Connector1/2(M30_rtu_data)
  RFID_rtu/3(XGCS49 0 1201_rtu_data) -> 5 pin Male M12 Connector1/3(XGCS49 0 1201_rtu_data)
  RFID_rtu/4(XGCS 89 01201 _rtu_data) -> 5 pin Male M12 Connector1/4(XGCS49 0 B201 _rtu_data)
  RFID_rtu/6(XGCS49 L B201 _rtu_data) -> 5 pin Male M12 Connector1/5(XGCS49 L B201 _rtu_data)
  RFID_rtu/5(XGCS49 0 B201 _rtu_data) -> 5 pin Male M12 Connector1/6(XGCS 89 01201 _rtu_data)
  5 pin Male M12 Connector1/1(M18_rtu_data_2_ethernet_box) -> "XGSZ 84 EIP "/1(M18_rtu_data_2_ethernet_box)
  5 pin Male M12 Connector1/2(M30_rtu_data_2_ethernet_box) -> "XGSZ 84 EIP "/2(M30_rtu_data_2_ethernet_box)
  5 pin Male M12 Connector1/3(XGCS49 0 1201_rtu_data_2_ethernet_box) -> "XGSZ 84 EIP "/3(XGCS49 0 1201_rtu_data_2_ethernet_box)
  5 pin Male M12 Connector1/4(XGCS49 0 B201 _rtu_data_2_ethernet_box) -> "XGSZ 84 EIP "/4(XGCS49 0 B201 _rtu_data_2_ethernet_box)
  5 pin Male M12 Connector1/5(XGCS49 L B201 _rtu_data_2_ethernet_box) -> "XGSZ 84 EIP "/5(XGCS49 L B201 _rtu_data_2_ethernet_box)
  5 pin Male M12 Connector1/6(XGCS 89 01201 _rtu_data_2_ethernet_box) -> "XGSZ 84 EIP "/6(XGCS 89 01201 _rtu_data_2_ethernet_box)
  RFID_rtu2/1(M18_rtu_data) -> 5 pin Male M12 Connector2/1(M18_rtu_data)
  RFID_rtu2/2(M30_rtu_data) -> 5 pin Male M12 Connector2/2(M30_rtu_data)
  RFID_rtu2/3(XGCS49 0 1201_rtu_data) -> 5 pin Male M12 Connector2/3(XGCS49 0 1201_rtu_data)
  RFID_rtu2/4(XGCS 89 01201 _rtu_data) -> 5 pin Male M12 Connector2/4(XGCS49 0 B201 _rtu_data)
  RFID_rtu2/5(XGCS49 0 B201 _rtu_data) -> 5 pin Male M12 Connector2/5(XGCS49 L B201 _rtu_data)
  RFID_rtu2/6(XGCS49 L B201 _rtu_data) -> 5 pin Male M12 Connector2/6(XGCS 89 01201 _rtu_data)
  5 pin Male M12 Connector2/1(M18_rtu_data_2_modbus_ box) -> "XGSZ 84 ETH "/1(M18_rtu_data_2_modbus_ box)
  5 pin Male M12 Connector2/2(M30_rtu_data_2_modbus_box) -> "XGSZ 84 ETH "/2(M30_rtu_data_2_modbus_box)
  5 pin Male M12 Connector2/3(XGCS49 0 1201_rtu_data_2_modbus_box) -> "XGSZ 84 ETH "/3(XGCS49 0 1201_rtu_data_2_modbus_box)
  5 pin Male M12 Connector2/4(XGCS49 0 B201 _rtu_data_2_modbus_box) -> "XGSZ 84 ETH "/4(XGCS49 0 B201 _rtu_data_2_modbus_box)
  5 pin Male M12 Connector2/5(XGCS49 L B201 _rtu_data_2_modbus_box) -> "XGSZ 84 ETH "/5(XGCS49 L B201 _rtu_data_2_modbus_box)
  5 pin Male M12 Connector2/6(XGCS 89 01201 _rtu_data_2_modbus_box) -> "XGSZ 84 ETH "/6(XGCS 89 01201 _rtu_data_2_modbus_box)
  RFID_Modbus/1(XGCS 850C 201_ModusTCp_Data) -> M12 to RJ45/1(XGCS 850C 201_ModusTCp_Data)
  M12 to RJ45/1("    ") -> ModbusTCP_Network/2(XGCS 850C 201_ModusTCp_Data_2_network)
  M12 to RJ1/1(XGCS 850C 201_Ethernetp_Data_2_swtich) -> TCSESU051F0/3(XGCS 850C 201_Ethernetp_Data_2_swtich)
  RFID_Profinet/1(XGCS 850C 201_Profinet_Data) -> M12 to RJ2/1(XGCS 850C 201_Profinet_Data)
  M12 to RJ2/1(XGCS 850C 201_Profinet_Data_2_network) -> Profinet_network/3(XGCS 850C 201_Profinet_Data)

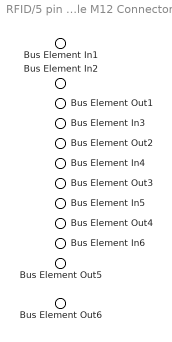
== system RFID/5 pin Male M12 Connector ==
  Bus Element In1 : Inport  PortName=M18_rtu_data
  Bus Element In2 : Inport  Port=2  PortName=M30_rtu_data
  Bus Element In3 : Inport  Port=3  PortName=XGCS49 0 1201_rtu_data
  Bus Element In4 : Inport  Port=4  PortName=XGCS49 0 B201 _rtu_data
  Bus Element In5 : Inport  Port=5  PortName=XGCS49 L B201 _rtu_data
  Bus Element In6 : Inport  Port=6  PortName=XGCS 89 01201 _rtu_data
  Bus Element Out1 : Outport  PortName=M18_rtu_data_2_profinet_box
  Bus Element Out2 : Outport  Port=2  PortName=M30_rtu_data_2_profinet_box
  Bus Element Out3 : Outport  Port=3  PortName=XGCS49 0 1201_rtu_data_2_profinet_box
  Bus Element Out4 : Outport  Port=4  PortName=XGCS49 0 B201 _rtu_data_2_profinet_box
  Bus Element Out5 : Outport  Port=5  PortName=XGCS49 L B201 _rtu_data_2_profinet_box
  Bus Element Out6 : Outport  Port=6  PortName=XGCS 89 01201 _rtu_data_2_profinet_box

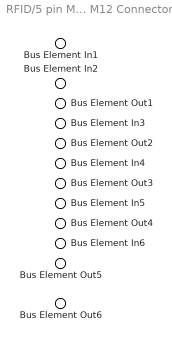
== system RFID/5 pin Male M12 Connector1 ==
  Bus Element In1 : Inport  PortName=M18_rtu_data
  Bus Element In2 : Inport  Port=2  PortName=M30_rtu_data
  Bus Element In3 : Inport  Port=3  PortName=XGCS49 0 1201_rtu_data
  Bus Element In4 : Inport  Port=4  PortName=XGCS49 0 B201 _rtu_data
  Bus Element In5 : Inport  Port=5  PortName=XGCS49 L B201 _rtu_data
  Bus Element In6 : Inport  Port=6  PortName=XGCS 89 01201 _rtu_data
  Bus Element Out1 : Outport  PortName=M18_rtu_data_2_ethernet_box
  Bus Element Out2 : Outport  Port=2  PortName=M30_rtu_data_2_ethernet_box
  Bus Element Out3 : Outport  Port=3  PortName=XGCS49 0 1201_rtu_data_2_ethernet_box
  Bus Element Out4 : Outport  Port=4  PortName=XGCS49 0 B201 _rtu_data_2_ethernet_box
  Bus Element Out5 : Outport  Port=5  PortName=XGCS49 L B201 _rtu_data_2_ethernet_box
  Bus Element Out6 : Outport  Port=6  PortName=XGCS 89 01201 _rtu_data_2_ethernet_box

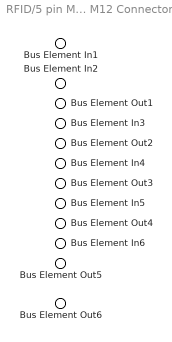
== system RFID/5 pin Male M12 Connector2 ==
  Bus Element In1 : Inport  PortName=M18_rtu_data
  Bus Element In2 : Inport  Port=2  PortName=M30_rtu_data
  Bus Element In3 : Inport  Port=3  PortName=XGCS49 0 1201_rtu_data
  Bus Element In4 : Inport  Port=4  PortName=XGCS49 0 B201 _rtu_data
  Bus Element In5 : Inport  Port=5  PortName=XGCS49 L B201 _rtu_data
  Bus Element In6 : Inport  Port=6  PortName=XGCS 89 01201 _rtu_data
  Bus Element Out1 : Outport  PortName=M18_rtu_data_2_modbus_ box
  Bus Element Out2 : Outport  Port=2  PortName=M30_rtu_data_2_modbus_box
  Bus Element Out3 : Outport  Port=3  PortName=XGCS49 0 1201_rtu_data_2_modbus_box
  Bus Element Out4 : Outport  Port=4  PortName=XGCS49 0 B201 _rtu_data_2_modbus_box
  Bus Element Out5 : Outport  Port=5  PortName=XGCS49 L B201 _rtu_data_2_modbus_box
  Bus Element Out6 : Outport  Port=6  PortName=XGCS 89 01201 _rtu_data_2_modbus_box

== system RFID/5 pin-1 male connector M12 ==
  Bus Element In1 : Inport  PortName=XGCS49 1 B201_PNP_Data
  Bus Element Out1 : Outport  PortName=Descrete/Analog Input

== system RFID/CONTROL PC ==
  Bus Element Out1 : Outport  PortName=PLC_Programmation

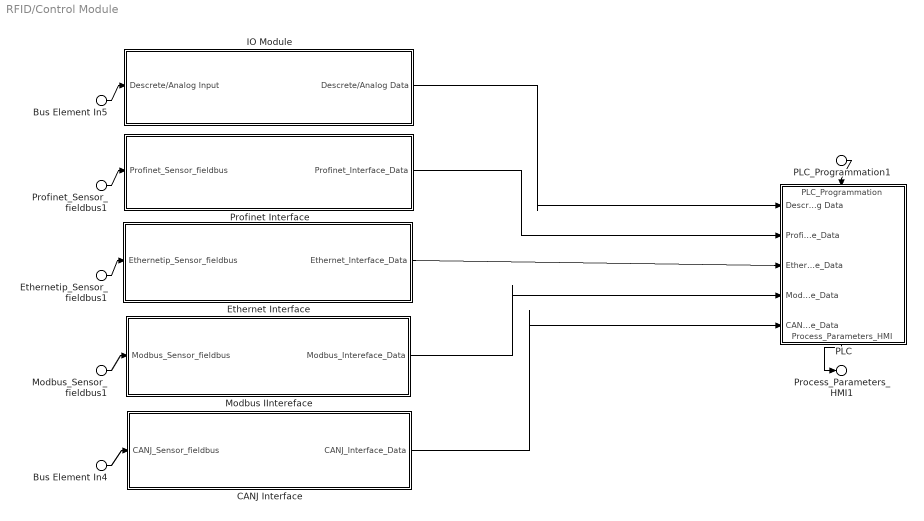
== system RFID/Control Module ==
  PLC_Programmation1 : Inport  PortName=PLC_Programmation
  Profinet_Sensor_fieldbus1 : Inport  Port=2  PortName=Profinet_Sensor_fieldbus
  Ethernetip_Sensor_fieldbus1 : Inport  Port=3  PortName=Ethernetip_Sensor_fieldbus
  Bus Element In4 : Inport  Port=4  PortName=CANJ_Sensor_fieldbus
  Bus Element In5 : Inport  Port=5  PortName=Descrete/Analog Input
  Modbus_Sensor_fieldbus1 : Inport  Port=6  PortName=Modbus_Sensor_fieldbus
  CANJ Interface : Subsystem
      settings: PortSchema="{\"entries\":[{\"content\":{\"headerSize\":26,\"margin\":15,\"minimumSpacing\":25,\"sides\":[{\"content\":{\"connectorIds\":[\"In1\"]},\"type\":\"ConnectorPlacement.EquallySpacedRectSide\",\"uuid\":\"ff8f3bf2-d6f6-4ecc-9677-a0e5f5ade440\"},{\"content\":{\"connectorIds\":[\"Out1\"],\"side\":\"RIGHT\"},\"type\":\"ConnectorPlacement.EquallySpacedRectSide\",\"uuid\":\"fe155757-f3d5-40d8-a583-dbbc24843437\"},{\"content\":{\"side\":\"TOP\"},\"type\":\"ConnectorPlacement.EquallySpacedRectSide\",\"uuid\":\"51bc4fd0-0675-45de-93bd-0dc8d94c5489\"}]},\"type\":\"ConnectorPlacement.EquallySpacedConnector\",\"uuid\":\"7eb8fdf8-dbe2-49f3-b9bd-384f85dcc997\"}],\"packageUris\":[\"http://schema.mathworks.com/mf0/Connector/R2020b\"],\"version\":\"1.0\"}"
  Ethernet Interface : Subsystem
      settings: PortSchema="{\"entries\":[{\"content\":{\"headerSize\":26,\"margin\":15,\"minimumSpacing\":25,\"sides\":[{\"content\":{\"connectorIds\":[\"In1\"]},\"type\":\"ConnectorPlacement.EquallySpacedRectSide\",\"uuid\":\"ff8f3bf2-d6f6-4ecc-9677-a0e5f5ade440\"},{\"content\":{\"connectorIds\":[\"Out1\"],\"side\":\"RIGHT\"},\"type\":\"ConnectorPlacement.EquallySpacedRectSide\",\"uuid\":\"fe155757-f3d5-40d8-a583-dbbc24843437\"},{\"content\":{\"side\":\"TOP\"},\"type\":\"ConnectorPlacement.EquallySpacedRectSide\",\"uuid\":\"51bc4fd0-0675-45de-93bd-0dc8d94c5489\"}]},\"type\":\"ConnectorPlacement.EquallySpacedConnector\",\"uuid\":\"7eb8fdf8-dbe2-49f3-b9bd-384f85dcc997\"}],\"packageUris\":[\"http://schema.mathworks.com/mf0/Connector/R2020b\"],\"version\":\"1.0\"}"
  IO Module : Subsystem
      settings: PortSchema="{\"entries\":[{\"content\":{\"headerSize\":26,\"margin\":15,\"minimumSpacing\":25,\"sides\":[{\"content\":{\"connectorIds\":[\"In1\"]},\"type\":\"ConnectorPlacement.EquallySpacedRectSide\",\"uuid\":\"ff8f3bf2-d6f6-4ecc-9677-a0e5f5ade440\"},{\"content\":{\"connectorIds\":[\"Out1\"],\"side\":\"RIGHT\"},\"type\":\"ConnectorPlacement.EquallySpacedRectSide\",\"uuid\":\"fe155757-f3d5-40d8-a583-dbbc24843437\"},{\"content\":{\"side\":\"TOP\"},\"type\":\"ConnectorPlacement.EquallySpacedRectSide\",\"uuid\":\"51bc4fd0-0675-45de-93bd-0dc8d94c5489\"}]},\"type\":\"ConnectorPlacement.EquallySpacedConnector\",\"uuid\":\"7eb8fdf8-dbe2-49f3-b9bd-384f85dcc997\"}],\"packageUris\":[\"http://schema.mathworks.com/mf0/Connector/R2020b\"],\"version\":\"1.0\"}"
  Modbus IIntereface : Subsystem
      settings: PortSchema="{\"entries\":[{\"content\":{\"headerSize\":26,\"margin\":15,\"minimumSpacing\":25,\"sides\":[{\"content\":{\"connectorIds\":[\"In1\"]},\"type\":\"ConnectorPlacement.EquallySpacedRectSide\",\"uuid\":\"ff8f3bf2-d6f6-4ecc-9677-a0e5f5ade440\"},{\"content\":{\"connectorIds\":[\"Out1\"],\"side\":\"RIGHT\"},\"type\":\"ConnectorPlacement.EquallySpacedRectSide\",\"uuid\":\"fe155757-f3d5-40d8-a583-dbbc24843437\"},{\"content\":{\"side\":\"TOP\"},\"type\":\"ConnectorPlacement.EquallySpacedRectSide\",\"uuid\":\"51bc4fd0-0675-45de-93bd-0dc8d94c5489\"}]},\"type\":\"ConnectorPlacement.EquallySpacedConnector\",\"uuid\":\"7eb8fdf8-dbe2-49f3-b9bd-384f85dcc997\"}],\"packageUris\":[\"http://schema.mathworks.com/mf0/Connector/R2020b\"],\"version\":\"1.0\"}"
  PLC : Subsystem
      settings: PortSchema="{\"entries\":[{\"content\":{\"headerSize\":26,\"margin\":15,\"minimumSpacing\":25,\"sides\":[{\"content\":{\"connectorIds\":[\"In1\",\"In4\",\"In5\",\"In6\",\"In2\"]},\"type\":\"ConnectorPlacement.EquallySpacedRectSide\",\"uuid\":\"ff8f3bf2-d6f6-4ecc-9677-a0e5f5ade440\"},{\"content\":{\"side\":\"RIGHT\"},\"type\":\"ConnectorPlacement.EquallySpacedRectSide\",\"uuid\":\"fe155757-f3d5-40d8-a583-dbbc24843437\"},{\"content\":{\"connectorIds\":[\"In3\"],\"side\":\"TOP\"},\"type\":\"ConnectorPlacement.EquallySpacedRectSide\",\"uuid\":\"51bc4fd0-0675-45de-93bd-0dc8d94c5489\"},{\"content\":{\"connectorIds\":[\"Out1\"],\"side\":\"BOTTOM\"},\"type\":\"ConnectorPlacement.EquallySpacedRectSide\",\"uuid\":\"b7b44f41-0e2c-4bbd-9aa1-2b70573de7d3\"}]},\"type\":\"ConnectorPlacement.EquallySpacedConnector\",\"uuid\":\"7eb8fdf8-dbe2-49f3-b9bd-384f85dcc997\"}],\"packageUris\":[\"http://schema.mathworks.com/mf0/Connector/R2020b\"],\"version\":\"1.0\"}"
  Profinet Interface : Subsystem
      settings: PortSchema="{\"entries\":[{\"content\":{\"headerSize\":26,\"margin\":15,\"minimumSpacing\":25,\"sides\":[{\"content\":{\"connectorIds\":[\"In1\"]},\"type\":\"ConnectorPlacement.EquallySpacedRectSide\",\"uuid\":\"ff8f3bf2-d6f6-4ecc-9677-a0e5f5ade440\"},{\"content\":{\"connectorIds\":[\"Out1\"],\"side\":\"RIGHT\"},\"type\":\"ConnectorPlacement.EquallySpacedRectSide\",\"uuid\":\"fe155757-f3d5-40d8-a583-dbbc24843437\"},{\"content\":{\"side\":\"TOP\"},\"type\":\"ConnectorPlacement.EquallySpacedRectSide\",\"uuid\":\"51bc4fd0-0675-45de-93bd-0dc8d94c5489\"}]},\"type\":\"ConnectorPlacement.EquallySpacedConnector\",\"uuid\":\"7eb8fdf8-dbe2-49f3-b9bd-384f85dcc997\"}],\"packageUris\":[\"http://schema.mathworks.com/mf0/Connector/R2020b\"],\"version\":\"1.0\"}"
  Process_Parameters_HMI1 : Outport  PortName=Process_Parameters_HMI
  wires:
  Modbus_Sensor_fieldbus1/1 -> Modbus IIntereface/1(Modbus_Sensor_fieldbus)
  Profinet_Sensor_fieldbus1/1 -> Profinet Interface/1(Profinet_Sensor_fieldbus)
  Ethernetip_Sensor_fieldbus1/1 -> Ethernet Interface/1(Ethernetip_Sensor_fieldbus)
  Profinet Interface/1(Profinet_Interface_Data) -> PLC/4(Profinet_Interface_Data)
  Modbus IIntereface/1(Modbus_Intereface_Data) -> PLC/6(Modbus_Intereface_Data)
  PLC/1(Process_Parameters_HMI) -> Process_Parameters_HMI1/1
  Ethernet Interface/1(Ethernet_Interface_Data) -> PLC/5(Ethernet_Interface_Data)
  PLC_Programmation1/1 -> PLC/3(PLC_Programmation)
  CANJ Interface/1(CANJ_Interface_Data) -> PLC/2(CANJ_Interface_Data)
  Bus Element In4/1 -> CANJ Interface/1(CANJ_Sensor_fieldbus)
  IO Module/1(Descrete/Analog Data) -> PLC/1(Descrete/Analog Data)
  Bus Element In5/1 -> IO Module/1(Descrete/Analog Input)

== system RFID/Deutsch 6-pin Connector ==
  Bus Element In1 : Inport  PortName=XGCS460B201_CANJ_Data
  Bus Element Out1 : Outport  PortName=CANJ_Sensor_fieldbus

== system RFID/EthernetIP_network ==
  Bus Element In1 : Inport  PortName=ethernet ip data
  Bus Element Out1 : Outport  PortName=Ethernetip_Sensor_fieldbus

== system RFID/HMI ==
  Bus Element In1 : Inport  PortName=Process_Parameters_HMI

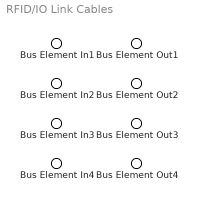
== system RFID/IO Link Cables ==
  Bus Element In1 : Inport  PortName=XGCS 89 01201_IOLimk_data
  Bus Element In2 : Inport  Port=2  PortName=XGCS 49 01201_IOLink_data
  Bus Element In3 : Inport  Port=3  PortName=M18_IOLink_data
  Bus Element In4 : Inport  Port=4  PortName=M30_IOLink_data
  Bus Element Out1 : Outport  PortName=XGCS 89 01201_IOLimk_data_2_master
  Bus Element Out2 : Outport  Port=2  PortName=XGCS 49 01201_IOLink_data_2_master
  Bus Element Out3 : Outport  Port=3  PortName=M18_IOLink_data_2_master
  Bus Element Out4 : Outport  Port=4  PortName=M30_IOLink_data_2_masters

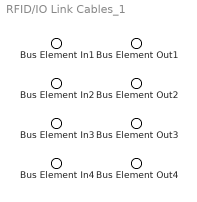
== system RFID/IO Link Cables_1 ==
  Bus Element In1 : Inport  PortName=XGCS 89 01201_IOLimk_data
  Bus Element In2 : Inport  Port=2  PortName=XGCS 49 01201_IOLink_data
  Bus Element In3 : Inport  Port=3  PortName=M18_IOLink_data
  Bus Element In4 : Inport  Port=4  PortName=M30_IOLink_data
  Bus Element Out1 : Outport  PortName=XGCS 89 01201_IOLimk_data_2_master
  Bus Element Out2 : Outport  Port=2  PortName=XGCS 49 01201_IOLink_data_2_master
  Bus Element Out3 : Outport  Port=3  PortName=M18_IOLink_data_2_master
  Bus Element Out4 : Outport  Port=4  PortName=M30_IOLink_data_2_masters

== system RFID/IOLink_master_EthernetIP ==
  Bus Element In1 : Inport  PortName=XGCS 49 01201_IOLink_data
  Bus Element In2 : Inport  Port=2  PortName=XGCS 89 01201_IOLimk_data
  Bus Element In3 : Inport  Port=3  PortName=M18_IOLink_data
  Bus Element In4 : Inport  Port=4  PortName=M30_IOLink_data
  Bus Element Out1 : Outport  PortName=IOLink_master_Profinet_serial_data_EthernetIP

== system RFID/IOLink_master_Profinet ==
  Bus Element In1 : Inport  PortName=XGCS 89 01201_IOLimk_data_2_master
  Bus Element In2 : Inport  Port=2  PortName=XGCS 49 01201_IOLink_data_2_master
  Bus Element In3 : Inport  Port=3  PortName=M18_IOLink_data_2_master
  Bus Element In4 : Inport  Port=4  PortName=M30_IOLink_data_2_masters
  Bus Element Out1 : Outport  PortName=IOLink_master_Profinet_serial_data_profinet

== system RFID/M12 to RJ1 ==
  Bus Element In1 : Inport  PortName=XGCS 850C 201_Ethernetp_Data
  Bus Element Out1 : Outport  PortName=XGCS 850C 201_Ethernetp_Data_2_swtich

== system RFID/M12 to RJ2 ==
  Bus Element In1 : Inport  PortName=XGCS 850C 201_Profinet_Data
  Bus Element Out1 : Outport  PortName=XGCS 850C 201_Profinet_Data_2_network

== system RFID/M12 to RJ45 ==
  Bus Element In1 : Inport  PortName=XGCS 850C 201_ModusTCp_Data
  Bus Element Out1 : Outport  PortName=""

== system RFID/ModbusTCP_Network ==
  Bus Element In1 : Inport  PortName=XGSZ84 ETH _serial_data_Mobdus
  Bus Element In2 : Inport  Port=2  PortName=XGCS 850C 201_ModusTCp_Data_2_network
  Bus Element Out1 : Outport  PortName=Modbus_Sensor_fieldbus
